simulink model "Assemble_Blocks_Aug_24"  (R2019a)
settings: Solver=VariableStepAuto  StartTime=0.0  StopTime=10.0  RelTol=1e-3
libraries: sailbot_library x19
settings Model: Creator=tylerlum  LastModifiedBy=tylerlum

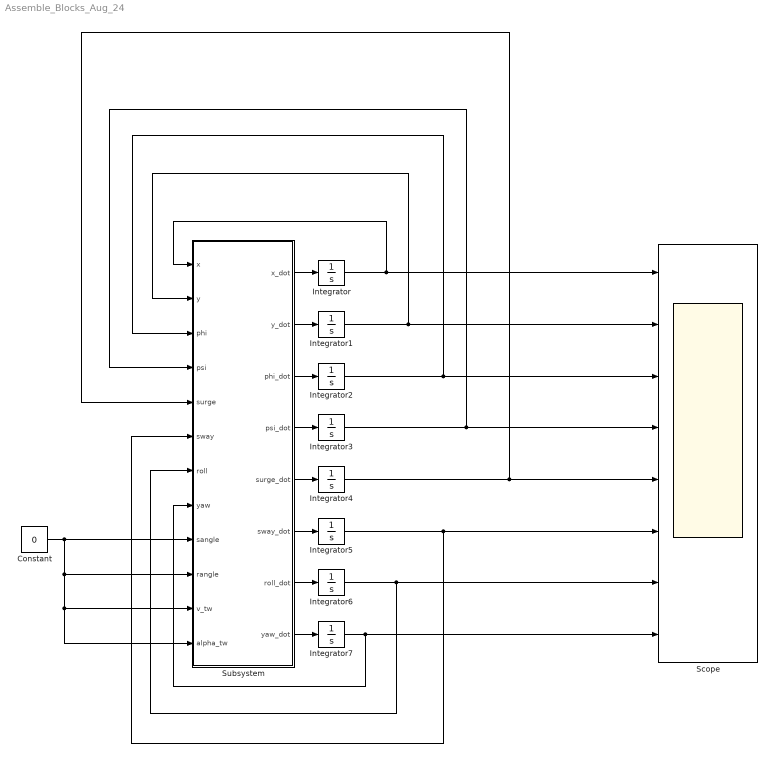
== system Assemble_Blocks_Aug_24 ==
  Constant : Constant  Value=0
  Integrator{,1..7} (8 alike) : Integrator
  Scope : Scope  NumInputPorts=8
  Subsystem : Subsystem
  wires:
  Subsystem/1(x_dot) -> Integrator/1
  Integrator/1 -> Scope/1, Subsystem/1(x)
  Subsystem/2(y_dot) -> Integrator1/1
  Subsystem/3(phi_dot) -> Integrator2/1
  Subsystem/4(psi_dot) -> Integrator3/1
  Subsystem/5(surge_dot) -> Integrator4/1
  Subsystem/6(sway_dot) -> Integrator5/1
  Subsystem/7(roll_dot) -> Integrator6/1
  Subsystem/8(yaw_dot) -> Integrator7/1
  Integrator1/1 -> Scope/2, Subsystem/2(y)
  Integrator2/1 -> Scope/3, Subsystem/3(phi)
  Integrator3/1 -> Scope/4, Subsystem/4(psi)
  Integrator7/1 -> Scope/8, Subsystem/8(yaw)
  Integrator6/1 -> Scope/7, Subsystem/7(roll)
  Integrator5/1 -> Scope/6, Subsystem/6(sway)
  Integrator4/1 -> Subsystem/5(surge), Scope/5
  Constant/1 -> Subsystem/10(rangle), Subsystem/11(v_tw), Subsystem/12(alpha_tw), Subsystem/9(sangle)

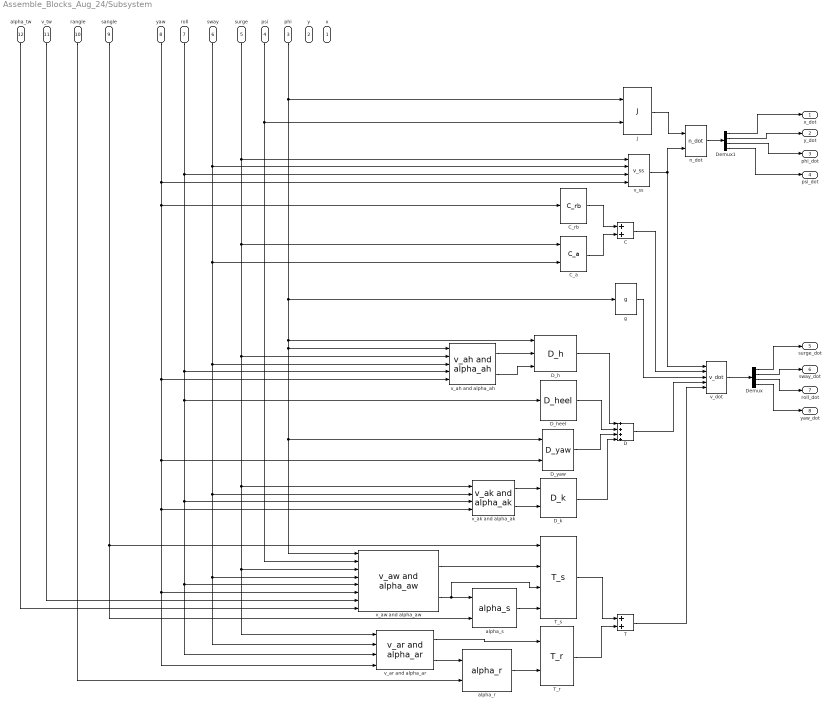
== system Assemble_Blocks_Aug_24/Subsystem ==
  x : Inport
  y : Inport  Port=2
  phi : Inport  Port=3
  psi : Inport  Port=4
  surge : Inport  Port=5
  sway : Inport  Port=6
  roll : Inport  Port=7
  yaw : Inport  Port=8
  sangle : Inport  Port=9
  rangle : Inport  Port=10
  v_tw : Inport  Port=11
  alpha_tw : Inport  Port=12
  C : Sum
  C_a : sailbot_library/C_a  SystemSampleTime=-1
  C_rb : sailbot_library/C_rb  SystemSampleTime=-1
  D : Sum  Inputs=4
  D_h : sailbot_library/D_h  SystemSampleTime=-1
  "D_heel " : sailbot_library/D_heel   SystemSampleTime=-1
  D_k : sailbot_library/D_k  SystemSampleTime=-1
  D_yaw : sailbot_library/D_yaw  SystemSampleTime=-1
  Demux : Demux
  Demux1 : Demux
  J : sailbot_library/J  SystemSampleTime=-1
  T : Sum
  T_r : sailbot_library/T_r  SystemSampleTime=-1
  "T_s " : sailbot_library/T_s   SystemSampleTime=-1
  alpha_r : sailbot_library/alpha_r  SystemSampleTime=-1
  alpha_s : sailbot_library/alpha_s  SystemSampleTime=-1
  g : sailbot_library/g  SystemSampleTime=-1
  n_dot : sailbot_library/n_dot  SystemSampleTime=-1
  v_ah and alpha_ah : sailbot_library/v_ah and alpha_ah  SystemSampleTime=-1
  v_ak and alpha_ak : sailbot_library/v_ak and alpha_ak  SystemSampleTime=-1
  v_ar and alpha_ar : sailbot_library/v_ar and alpha_ar  SystemSampleTime=-1
  v_aw and alpha_aw : sailbot_library/v_aw and alpha_aw  SystemSampleTime=-1
  v_dot : sailbot_library/v_dot  SystemSampleTime=-1
  v_ss : sailbot_library/v_ss  SystemSampleTime=-1
  x_dot : Outport
  y_dot : Outport  Port=2
  phi_dot : Outport  Port=3
  psi_dot : Outport  Port=4
  surge_dot : Outport  Port=5
  sway_dot : Outport  Port=6
  roll_dot : Outport  Port=7
  yaw_dot : Outport  Port=8
  wires:
  alpha_s/1 -> "T_s "/4
  Demux/4 -> yaw_dot/1
  "T_s "/1 -> T/1
  C/1 -> v_dot/2
  D_yaw/1 -> D/3
  v_ah and alpha_ah/1 -> D_h/2
  D/1 -> v_dot/4
  v_aw and alpha_aw/1 -> "T_s "/2
  v_ak and alpha_ak/1 -> D_k/1
  v_ak and alpha_ak/2 -> D_k/2
  Demux/3 -> roll_dot/1
  C_a/1 -> C/2
  J/1 -> n_dot/1
  D_k/1 -> D/4
  psi/1 -> v_aw and alpha_aw/2, J/2
  Demux1/4 -> psi_dot/1
  Demux1/2 -> y_dot/1
  T/1 -> v_dot/5
  v_aw and alpha_aw/2 -> "T_s "/3, alpha_s/1
  alpha_tw/1 -> v_aw and alpha_aw/8
  sway/1 -> v_ss/2, C_a/2, v_ah and alpha_ah/3, v_aw and alpha_aw/4, v_ar and alpha_ar/2, v_ak and alpha_ak/2
  alpha_r/1 -> T_r/2
  v_tw/1 -> v_aw and alpha_aw/7
  D_h/1 -> D/1
  g/1 -> v_dot/3
  C_rb/1 -> C/1
  v_ah and alpha_ah/2 -> D_h/3
  v_ss/1 -> v_dot/1, n_dot/2
  n_dot/1 -> Demux1/1
  Demux1/3 -> phi_dot/1
  surge/1 -> v_ak and alpha_ak/1, v_aw and alpha_aw/3, v_ar and alpha_ar/1, v_ah and alpha_ah/2, C_a/1, v_ss/1
  Demux1/1 -> x_dot/1
  v_ar and alpha_ar/1 -> T_r/1
  "D_heel "/1 -> D/2
  rangle/1 -> alpha_r/2
  yaw/1 -> v_ss/4, D_yaw/2, v_ak and alpha_ak/4, v_ar and alpha_ar/4, v_aw and alpha_aw/6, v_ah and alpha_ah/5, C_rb/1
  phi/1 -> J/1, D_h/1, D_yaw/1, v_aw and alpha_aw/1, v_ah and alpha_ah/1, g/1
  Demux/1 -> surge_dot/1
  sangle/1 -> "T_s "/1, alpha_s/2
  v_ar and alpha_ar/2 -> alpha_r/1
  T_r/1 -> T/2
  Demux/2 -> sway_dot/1
  roll/1 -> v_ss/3, v_ah and alpha_ah/4, "D_heel "/1, v_ak and alpha_ak/3, v_aw and alpha_aw/5, v_ar and alpha_ar/3
  v_dot/1 -> Demux/1
